simulink model "zad_hamsam"  (R2013a)
settings: Solver=ode4  StartTime=0.0  StopTime=50.0  FixedStep=0.001  RelTol=1e-3
values from neighbouring files (symbols this model uses):
  h = 40    [2.mat]    (also in 3.mat)
  k1 = 6000    [1.mat]    (also in 2.mat = 55000; 3.mat = 55000)
  k2 = 300000    [2.mat]    (also in 3.mat)
  m1 = 14000    [1.mat]    (also in 2.mat; 3.mat)
  m2 = 500    [2.mat]    (also in 3.mat)
  m3 = 200    [3.mat]
  v0 = 70    [1.mat]    (also in 2.mat; 3.mat = 67)
settings Model: Creator=student  LastModifiedBy=adasdeb
settings DataIOCC: MaxDataPoints=1000000  SignalLoggingSaveFormat=ModelDataLogs
settings OptimizationCC: ExpressionDepthLimit=2147483647
settings DebuggingCC: FcnCallInpInsideContextMsg=EnableAllAsWarning

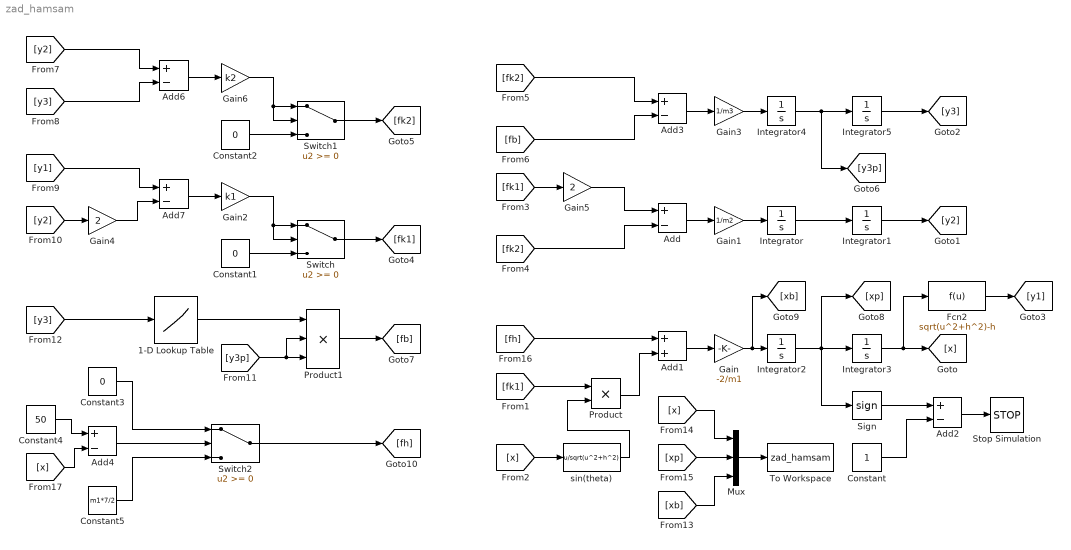
== system zad_hamsam ==
  1-D Lookup Table : Lookup_n-D  NumberOfTableDimensions=1  BreakpointsForDimension1=[0 10 20 30 40 50 60 70 80 90 94 98 102 104 107 120]  Table=[833 400 160 320 520 520 660 830 1070 1600 2100 2800 4100 5000 9000 9000]  RndMeth=Simplest  InputSameDT=on
  Add{,2..4,6..7} (6 alike) : Sum  Inputs=+-
  Add1 : Sum
  Constant : Constant
  Constant1 : Constant  Value=0
  Constant2 : Constant  Value=0
  Constant3 : Constant  Value=0
  Constant4 : Constant  Value=50
  Constant5 : Constant  Value=m1*7/2
  Fcn2 : Fcn  Expr=sqrt(u^2+h^2)-h
  Gain : Gain  Gain=-2/m1
  Gain1 : Gain  Gain=1/m2
  Gain2 : Gain  Gain=k1
  Gain3 : Gain  Gain=1/m3
  Gain4 : Gain  Gain=2
  Gain5 : Gain  Gain=2
  Gain6 : Gain  Gain=k2
  Integrator{,1,3..5} (5 alike) : Integrator
  Integrator2 : Integrator  InitialCondition=v0
  Mux : Mux  Inputs=3
  Product : Product  RndMeth=Zero
  Product1 : Product  Inputs=3  RndMeth=Zero
  Sign : Signum
  Stop Simulation : Stop
  Switch : Switch
  Switch1 : Switch
  Switch2 : Switch
  To Workspace : ToWorkspace  VariableName=zad_hamsam  SampleTime=-1
  sin(theta) : Fcn  Expr=u/sqrt(u^2+h^2)
  wires:
  Integrator/1 -> Integrator1/1
  Gain1/1 -> Integrator/1
  Add/1 -> Gain1/1
  Integrator3/1 -> Fcn2/1, [x]
  Integrator2/1 -> Sign/1, [xp], Integrator3/1
  Integrator1/1 -> [y2]
  Integrator4/1 -> [y3p], Integrator5/1
  Gain3/1 -> Integrator4/1
  Add3/1 -> Gain3/1
  Integrator5/1 -> [y3]
  Fcn2/1 -> [y1]
  Constant1/1 -> Switch/3
  Constant2/1 -> Switch1/3
  Gain6/1 -> Switch1/2, Switch1/1
  Add6/1 -> Gain6/1
  [y3] -> Add6/2
  [y2] -> Add6/1
  Gain2/1 -> Switch/2, Switch/1
  Add7/1 -> Gain2/1
  [y1] -> Add7/1
  [y2] -> Gain4/1
  Gain4/1 -> Add7/2
  Switch1/1 -> [fk2]
  Switch/1 -> [fk1]
  [x] -> sin(theta)/1
  [fk2] -> Add/2
  Gain5/1 -> Add/1
  [fk1] -> Gain5/1
  [fk2] -> Add3/1
  [fb] -> Add3/2
  Product1/1 -> [fb]
  1-D Lookup Table/1 -> Product1/1
  [y3p] -> Product1/2, Product1/3
  [y3] -> 1-D Lookup Table/1
  Sign/1 -> Add2/1
  Constant/1 -> Add2/2
  Add2/1 -> Stop Simulation/1
  Add4/1 -> Switch2/2
  [x] -> Add4/2
  Constant4/1 -> Add4/1
  Constant5/1 -> Switch2/3
  Constant3/1 -> Switch2/1
  Switch2/1 -> [fh]
  Gain/1 -> [xb], Integrator2/1
  Add1/1 -> Gain/1
  [fh] -> Add1/1
  Mux/1 -> To Workspace/1
  [xb] -> Mux/3
  [xp] -> Mux/2
  [x] -> Mux/1
  Product/1 -> Add1/2
  [fk1] -> Product/1
  sin(theta)/1 -> Product/2
